simulink model "Appl_PaMemory_CtrlModel"  (R2018b)
settings: configuration reference "CodeConfig_10_ms" (kept outside this file)
undefined symbols (not defined in the file): CAL_PaMem_100MS, CAL_PaMem_90MS, D_ToleranceDistance, FALSE, TRUE
libraries: DareLib x89, simulink x1
(part 3 of 3)

== stateflow chart Appl_PaMemory_CtrlModel/LogicCtrl/LocalAdjustCtrl/MemoryCall ==
  state MemoryCallLogic [parallel]
    settings: executionOrder=1
    state MemoryCallInactive
      en:
      MemoryCallFbSts = enMemCallFb.EN_MemCallFb_NULL;
      MemoryButtonNum = 0;
      MsgSendFinishedFlag = FALSE;
      SeatMemoryValidReq = FALSE;
      SeatHeightPosiReq = 0;
      SeatLengthPosiReq = 0;
      SeatBackPosiReq = 0;
      SeatFrontPosiReq = 0;
    state MemoryCallActive
      state Wait
        (default) -> (junction 52)
        Wait -> (junction 52) [order 1]
        (junction 52) -> (junction 55)
        (junction 55) -> (junction 57) [order 1] : /*获取记忆调用1目标位置*/
            | [SeatMemBtn == enMemBtn.EN_MemBtn_Call1]
        (junction 55) -> (junction 63) [order 2]
        (junction 57) -> (junction 59) : {MemoryButtonNum = 1;
            | SeatMemoryValidReq = MemoryValid;
            | SeatHeightPosiReq = MemoryHeightPosi;
            | SeatLengthPosiReq = MemoryLengthPosi;
            | SeatBackPosiReq = MemoryBackPosi;
            | SeatFrontPosiReq = MemoryFrontPosi;}
        (junction 59) -> (junction 63)
        (junction 63) -> (junction 67)
        (junction 67) -> (junction 69) [order 1] : /*获取记忆调用2目标位置*/
            | [SeatMemBtn == enMemBtn.EN_MemBtn_Call2]
        (junction 67) -> (junction 73) [order 2]
        (junction 69) -> (junction 71) : {MemoryButtonNum = 2;
            | SeatMemoryValidReq = MemoryValid;
            | SeatHeightPosiReq = MemoryHeightPosi;
            | SeatLengthPosiReq = MemoryLengthPosi;
            | SeatBackPosiReq = MemoryBackPosi;
            | SeatFrontPosiReq = MemoryFrontPosi;}
        (junction 71) -> (junction 73)
        (junction 73) -> (junction 76)
        (junction 76) -> (junction 78) [order 1] : /*获取记忆调用3目标位置*/
            | [SeatMemBtn == enMemBtn.EN_MemBtn_Call3]
        (junction 76) -> (junction 82) [order 2]
        (junction 78) -> (junction 80) : {MemoryButtonNum = 3;
            | SeatMemoryValidReq = MemoryValid;
            | SeatHeightPosiReq = MemoryHeightPosi;
            | SeatLengthPosiReq = MemoryLengthPosi;
            | SeatBackPosiReq = MemoryBackPosi;
            | SeatFrontPosiReq = MemoryFrontPosi;}
        (junction 80) -> (junction 82)
        (junction 82) -> (junction 85)
        (junction 85) -> (junction 126) [order 1] : /* 调用不满足 停止电机运动 */
            | [MemCallPC_Flag == FALSE || SeatMemoryValidReq == FALSE]
        (junction 85) -> (junction 131) [order 2] : {MemoryCallFbSts = enMemCallFb.EN_MemCallFb_Wait;}
        (junction 126) -> (junction 128) : {SeatMemoryValidReq = FALSE;
            | SeatHeightPosiReq = 0;
            | SeatLengthPosiReq = 0;
            | SeatBackPosiReq = 0;
            | SeatFrontPosiReq = 0;}
        (junction 128) -> (junction 131)
        (junction 131) -> (junction 133)
      state Succeed
        en:
        MemoryCallFbSts = enMemCallFb.EN_MemCallFb_Succeed;
        WaitTimeCnt = 0;
        //SetCanSendEvent(0x3B2);
        du:
        WaitTimeCnt += 1;
      state Fail
        en:
        MemoryCallFbSts = enMemCallFb.EN_MemCallFb_Faild;
        WaitTimeCnt = 0;
        //SetCanSendEvent(0x3B2);
        du:
        WaitTimeCnt += 1;
      state MessageSendFinish
        en:
        MsgSendFinishedFlag = TRUE;
        MemoryCallFbSts = enMemCallFb.EN_MemCallFb_NULL;
      note: /*如果服务层没有CAN反馈标志，使用延时90ms(20ms/5帧)*/
      (default) -> Wait
      Wait -> Succeed [order 4] : /*(高度自动运行成功标志位 == TRUE || 高度堵转)
          | && (纵向自动运行成功标志位 == TRUE || 纵向堵转)
          | && (靠背自动运行成功标志位 == TRUE || 靠背堵转)
          | && (前部自动运行成功标志位 == TRUE || 前部堵转)*/
          | [/*(PaMem_HeightAutoRunFlag == enSeatAutoRunSts.EN_SEAT_SUCCESS ...
          | || PaMem_HeightLockFault == TRUE) ...
          | && */(PaMem_LengthAutoRunFlag == enSeatAutoRunSts.EN_SEAT_SUCCESS ...
          |     || PaMem_LengthLockFault == TRUE) ...
          | && (PaMem_BackAutoRunFlag == enSeatAutoRunSts.EN_SEAT_SUCCESS ...
          |     || PaMem_BackLockFault == TRUE) /*...
          | && (PaMem_FrontAutoRunFlag == enSeatAutoRunSts.EN_SEAT_SUCCESS ...
          |     || PaMem_FrontLockFault == TRUE)*/]
      Wait -> MessageSendFinish [order 2] : /* 位置未记忆 */
          | [SeatMemoryValidReq == FALSE]
          | /MemCallStopReason = enMemStopCause.EN_MemStop_PosiError;
      Wait -> Fail [order 1] : /*记忆调用前置条件不满足*/
          | [MemCallPC_Flag == FALSE ]
          | /MemCallStopReason = PreMemCallStop;
      Wait -> Fail [order 3] : /*1.此处接口需要与调节模型确认返回值
          | 2.此跳转包含霍尔故障
          | 高度自动运行成功标志位 == FALSE
          | || 纵向自动运行成功标志位 == FALSE
          | || 靠背自动运行成功标志位 == FALSE
          | || 前部自动运行成功标志位 == FALSE
          | /MemCallStopReason = 0xC:enMotorRunError*/
          | [/*PaMem_HeightAutoRunFlag == enSeatAutoRunSts.EN_SEAT_FAIL ...
          | || */PaMem_LengthAutoRunFlag == enSeatAutoRunSts.EN_SEAT_FAIL ...
          | || PaMem_BackAutoRunFlag == enSeatAutoRunSts.EN_SEAT_FAIL/* ...
          | || PaMem_FrontAutoRunFlag == enSeatAutoRunSts.EN_SEAT_FAIL*/]
          | /MemCallStopReason = enMemStopCause.EN_MemStop_MotorRunErr;
      Succeed -> MessageSendFinish : /*Srvl_CAN反馈报文发送完成 || 延时90ms*/
          | [WaitTimeCnt >= 2 ...
          | && GetCanSendEvent() == TRUE]
      Fail -> MessageSendFinish : /*Srvl_CAN反馈报文发送完成 || 延时90ms*/
          | [WaitTimeCnt >= 2 ...
          | && GetCanSendEvent() == TRUE]
    (default) -> MemoryCallInactive
    MemoryCallInactive -> MemoryCallActive [order 1] : /*SeatMemBtn变为CallButton1*/
        | [hasChangedTo(SeatMemBtn,enMemBtn.EN_MemBtn_Call1)]
    MemoryCallInactive -> MemoryCallActive [order 2] : /*SeatMemBtn变为CallButton2*/
        | [hasChangedTo(SeatMemBtn,enMemBtn.EN_MemBtn_Call2)]
    MemoryCallInactive -> MemoryCallActive [order 3] : /*SeatMemBtn变为CallButton3*/
        | [hasChangedTo(SeatMemBtn,enMemBtn.EN_MemBtn_Call3)]
    MemoryCallActive -> MemoryCallInactive : [MsgSendFinishedFlag == TRUE]
  state [CallFB1,CallFB2,CallFB3] = MemCallWaitFBFunc(ButtonNum,FBSts) [function]
  state MemoryCallMessageFeedback [parallel]
    settings: executionOrder=2
    state MemoryCallDefaultFeedback
      en:
      SeatMem1StsFb = enMemCallFb.EN_MemCallFb_NULL;
      SeatMem2StsFb = enMemCallFb.EN_MemCallFb_NULL;
      SeatMem3StsFb = enMemCallFb.EN_MemCallFb_NULL;
    state MemoryCallResultFeedback
      state MemoryCallRun
        en:
        [SeatMem1StsFb,SeatMem2StsFb,SeatMem3StsFb] = MemCallWaitFBFunc(MemoryButtonNum,MemoryCallFbSts);
        du:
        [SeatMem1StsFb,SeatMem2StsFb,SeatMem3StsFb] = MemCallWaitFBFunc(MemoryButtonNum,MemoryCallFbSts);
      state MemoryCallMotorStop
        en:
        FbWaitTimeCnt = 0;
        [SeatMem1StsFb,SeatMem2StsFb,SeatMem3StsFb] = MemCallWaitFBFunc(MemoryButtonNum,MemoryCallFbSts);
        SetCanSendFRSeatMem1Sts(SeatMem1StsFb);
        SetCanSendFRSeatMem2Sts(SeatMem2StsFb);
        SetCanSendFRSeatMem3Sts(SeatMem3StsFb);
        SetCanSendEvent(0x3B2);
        du:
        FbWaitTimeCnt += 1;
      (default) -> MemoryCallRun
      MemoryCallRun -> MemoryCallMotorStop : /*记忆调用结束*/
          | [MemoryCallFbSts == enMemCallFb.EN_MemCallFb_Succeed ...
          | || MemoryCallFbSts == enMemCallFb.EN_MemCallFb_Faild]
    (default) -> MemoryCallDefaultFeedback
    MemoryCallDefaultFeedback -> MemoryCallResultFeedback [order 1] : /*记忆调用开始运行*/
        | [MemoryCallFbSts == enMemCallFb.EN_MemCallFb_Wait]
    MemoryCallDefaultFeedback -> MemoryCallMotorStop [order 2] : /*记忆调用直接结束*/
        | [MemoryCallFbSts == enMemCallFb.EN_MemCallFb_Succeed ...
        | || MemoryCallFbSts == enMemCallFb.EN_MemCallFb_Faild]
    MemoryCallMotorStop -> MemoryCallDefaultFeedback : /*延时90ms*/
        | [FbWaitTimeCnt >= CAL_PaMem_90MS ...
        | || GetCanSendEvent() == TRUE]
  state SetCanSendEvent(In1) [function]
  state SetCanSendFRSeatMem1Sts(In1) [function]
  state SetCanSendFRSeatMem2Sts(In1) [function]
  state Out1 = GetCanSendEvent [function]
  state SetCanSendFRSeatMem3Sts(In1) [function]
  data: ButtonNum function_input; FBSts function_input; CallFB1 function_output; CallFB2 function_output; CallFB3 function_output; In1 function_input; In1 function_input; In1 function_input; Out1 function_output; In1 function_input; SeatMemoryValidReq output uint8; SeatHeightPosiReq output uint16; SeatLengthPosiReq output uint16; SeatBackPosiReq output uint16; SeatFrontPosiReq output uint16; MemCallStopReason output Enum: enMemStopCause; MemoryCallFbSts local Enum: enMemCallFb; MemoryButtonNum local Enum: enMemCallFb; MsgSendFinishedFlag local uint8; FALSE parameter; SeatMemBtn input; MemoryHeightPosi input; MemoryLengthPosi input; MemoryBackPosi input; MemoryFrontPosi input; MemoryValid input; PreMemCallStop input; PaMem_HeightAutoRunFlag input; PaMem_LengthAutoRunFlag input; PaMem_BackAutoRunFlag input; PaMem_FrontAutoRunFlag input; TRUE parameter; WaitTimeCnt local uint16; CAL_PaMem_90MS parameter; MemCallPC_Flag input; PaMem_HeightLockFault input; PaMem_LengthLockFault input; PaMem_BackLockFault input; PaMem_FrontLockFault input; SeatMem1StsFb output Enum: enMemCallFb; SeatMem2StsFb output Enum: enMemCallFb; SeatMem3StsFb output Enum: enMemCallFb; FbWaitTimeCnt local uint16

== stateflow chart Appl_PaMemory_CtrlModel/LogicCtrl/LocalAdjustCtrl/MemorySetLogic/FirstPosiMemSetFunc/FirstPosiMemSetFunc ==
  state MemoryHight(CurrentH) [function]
  state MemoryLength(CurrentL) [function]
  state MemoryBack(CurrentB) [function]
  state MemoryFront(CurrentF) [function]
  state MemoryValid(Sts) [function]
  (default) -> (junction 2)
  (junction 2) -> (junction 10)
  (junction 10) -> (junction 12) [order 1] : /* 记忆功能使能 */
      | [SeatMemCfg == TRUE]
  (junction 10) -> (junction 16) [order 2]
  (junction 12) -> (junction 14) : {MemoryHight(CurrentH);
      | MemoryLength(CurrentL);
      | MemoryBack(CurrentB);
      | MemoryFront(CurrentF);
      | MemoryValid(TRUE);}
  (junction 14) -> (junction 16)
  (junction 16) -> (junction 19)
  data: CurrentH function_input; CurrentL function_input; CurrentB function_input; CurrentF function_input; Sts function_input; SeatMemCfg input uint8; CurrentH input uint16; CurrentL input uint16; CurrentB input uint16; CurrentF input uint16; TRUE parameter

== stateflow chart Appl_PaMemory_CtrlModel/LogicCtrl/LocalAdjustCtrl/MemorySetLogic/SecondPosiMemSetFunc/SecondPosiMemSetFunc ==
  state MemoryHight(CurrentH) [function]
  state MemoryLength(CurrentL) [function]
  state MemoryBack(CurrentB) [function]
  state MemoryFront(CurrentF) [function]
  state MemoryValid(Sts) [function]
  (default) -> (junction 2)
  (junction 2) -> (junction 10)
  (junction 10) -> (junction 12) [order 1] : /* 记忆功能使能 */
      | [SeatMemCfg == TRUE]
  (junction 10) -> (junction 16) [order 2]
  (junction 12) -> (junction 14) : {MemoryHight(CurrentH);
      | MemoryLength(CurrentL);
      | MemoryBack(CurrentB);
      | MemoryFront(CurrentF);
      | MemoryValid(TRUE);}
  (junction 14) -> (junction 16)
  (junction 16) -> (junction 19)
  data: CurrentH function_input; CurrentL function_input; CurrentB function_input; CurrentF function_input; Sts function_input; SeatMemCfg input uint8; CurrentH input uint16; CurrentL input uint16; CurrentB input uint16; CurrentF input uint16; TRUE parameter

== stateflow chart Appl_PaMemory_CtrlModel/LogicCtrl/LocalAdjustCtrl/MemorySetLogic/ThirdPosiMemSetFunc/ThirdPosiMemSetFunc ==
  state MemoryHight(CurrentH) [function]
  state MemoryLength(CurrentL) [function]
  state MemoryBack(CurrentB) [function]
  state MemoryFront(CurrentF) [function]
  state MemoryValid(Sts) [function]
  (default) -> (junction 2)
  (junction 2) -> (junction 10)
  (junction 10) -> (junction 12) [order 1] : /* 记忆功能使能 */
      | [SeatMemCfg == TRUE]
  (junction 10) -> (junction 16) [order 2]
  (junction 12) -> (junction 14) : {MemoryHight(CurrentH);
      | MemoryLength(CurrentL);
      | MemoryBack(CurrentB);
      | MemoryFront(CurrentF);
      | MemoryValid(TRUE);}
  (junction 14) -> (junction 16)
  (junction 16) -> (junction 19)
  data: CurrentH function_input; CurrentL function_input; CurrentB function_input; CurrentF function_input; Sts function_input; SeatMemCfg input uint8; CurrentH input uint16; CurrentL input uint16; CurrentB input uint16; CurrentF input uint16; TRUE parameter

== stateflow chart Appl_PaMemory_CtrlModel/LogicCtrl/LocalAdjustCtrl/MemoryCall/MemCallWaitFBFunc/Chart ==
  (default) -> (junction 3)
  (junction 3) -> (junction 5) : {CallFB1 = enMemCallFb.EN_MemCallFb_NULL;
      | CallFB2 = enMemCallFb.EN_MemCallFb_NULL;
      | CallFB3 = enMemCallFb.EN_MemCallFb_NULL;}
  (junction 5) -> (junction 7) [order 1] : /* 调用位置1进行中 */
      | [ButtonNum == 1]
  (junction 5) -> (junction 14) [order 2]
  (junction 7) -> (junction 9) : {CallFB1 = FBSts;}
  (junction 14) -> (junction 16) [order 1] : /* 调用位置2 进行中 */
      | [ButtonNum == 2]
  (junction 14) -> (junction 20) [order 2] : {CallFB3 = FBSts;}
  (junction 16) -> (junction 18) : {CallFB2 = FBSts;}
  (junction 18) -> (junction 20)
  (junction 9) -> (junction 18)
  (junction 20) -> (junction 27)
  data: ButtonNum input uint8; FBSts input Enum: enMemCallFb; CallFB1 output Enum: enMemCallFb; CallFB2 output Enum: enMemCallFb; CallFB3 output Enum: enMemCallFb
